simulink model "OFDM_Tx_HW"  (R2020a)
settings: Solver=FixedStepDiscrete  StartTime=0.0  StopTime=inf  RelTol=1e-3
PostLoadFcn:
  | run ./scripts/filter_setup;
InitFcn:
  | % Set parameters
  | fs = 1e6;
  | 
  | % Load all required variables
  | load('variables/read_addr_data');
  | load('variables/read_addr_cp');
  | load('variables/read_addr_pream');
  | load('variables/read_addr_rx');
  | load('variables/pilot');
  | load('variables/sc_index');
  | load('variables/LTSfreq');
  | load('variables/STSfreq');
  | load('variables/LTSread');
  | load('variables/STSread');
  | 
  | run ./scripts/rfgen;
undefined symbols (not defined in the file): CIC_fine_Rx
libraries: hdlsllib x13, dspsigops x5, dspmlti4 x3, xbsIndex_r4 x1, lib_ofdmrx x1, lib_ofdmtx x1, dspobslib x1, lib_interpolatetx x1
settings Model: SimulationMode=accelerator  Creator=njb13206  LastModifiedBy=LDM
settings OptimizationCC: BlockReduction=off  ConditionallyExecuteInputs=off  DefaultParameterBehavior=Inlined
settings DebuggingCC: AlgebraicLoopMsg=error  IntegerOverflowMsg=none  ParameterPrecisionLossMsg=none  IntegerSaturationMsg=none
settings HardwareCC: ProdBitPerPointer=32  ProdBitPerSizeT=32  ProdBitPerPtrDiffT=32  ProdLargestAtomicFloat=None  ProdIntDivRoundTo=Undefined  ProdEndianess=Unspecified  ProdWordSize=32  ProdHWDeviceType=ASIC/FPGA->ASIC/FPGA  TargetBitPerPointer=64  TargetBitPerSizeT=64  TargetBitPerPtrDiffT=64  TargetLongLongMode=on  TargetIntDivRoundTo=Zero  TargetEndianess=LittleEndian  TargetWordSize=64  TargetHWDeviceType=Custom Processor->MATLAB Host Computer  ProdEqTarget=off

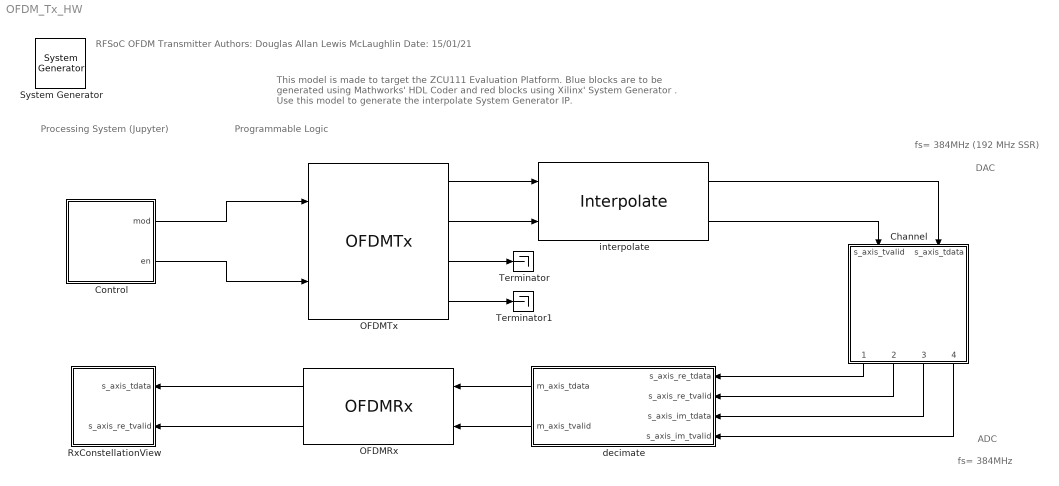
== system OFDM_Tx_HW ==
  note: This model is made to target the ZCU111 Evaluation Platform. Blue blocks are to be generated using Mathworks' HDL Coder and red blocks using Xilinx' System Generator .
      |
      | Use this model to generate the interpolate System Generator IP.
  note: Programmable Logic
  note: Processing System (Jupyter)
  note: DAC
  note: fs= 384MHz (192 MHz SSR)
  note: ADC
  note: fs= 384MHz
  note: RFSoC OFDM Transmitter
      | Authors: Douglas Allan
      | Lewis McLaughlin
      | Date: 15/01/21
  " System Generator" : xbsIndex_r4/ System Generator  Tag=genX  xilinxfamily=zynquplusRFSOC  part=xczu28dr  speed=-2-e  package=ffvg1517  synthesis_tool=Vivado  clock_wrapper=Clock Enables  directory=C:/Git/rfsoc_ofdm_workspace/models/sys_prj/tx  proj_type=Vivado  Synth_file=Vivado Synthesis Defaults  Impl_file=Vivado Implementation Defaults  testbench=off  simulink_period=1/192e6  sysclk_period=1000/192  dcm_input_clock_period=10  incr_netlist=off  trim_vbits=Everywhere in SubSystem  dbl_ovrd=According to Block Masks  core_generation=According to Block Masks  run_coregen=off  deprecated_control=off  eval_field=0  block_type=sysgen
  Channel : Subsystem
  Control : Subsystem  mask{mod_mask=512QAM, en=on}
      mask prompts: mod_mask "Modulation"; en "Enable"
      mask init:
      | % RF Signal Generator
      | if strcmpi(get_param(gcb, 'mod_mask'), 'BPSK')
      |     mod = 0;
      | elseif strcmpi(get_param(gcb, 'mod_mask'), 'QPSK')
      |     mod = 1;
      | elseif strcmpi(get_param(gcb, 'mod_mask'), '8PSK')
      |     mod = 2;
      | elseif strcmpi(get_param(gcb, 'mod_mask'), '16QAM')
      |     mod = 3;
      | elseif strcmpi(get_param(gcb, 'mod_mask'), '32QAM')
      |     mod = 4;
      | elseif strcmpi(get_param(gcb, 'mod_mask'), '64QAM')
      |     mod = 5;
      | elseif strcmpi(get_param(gcb, 'mod_mask'), '128QAM')
      |     mod = 6;
      | elseif strcmpi(get_param(gcb, 'mod_mask'), '256QAM')
      |     mod = 7;
      | elseif strcmpi(get_param(gcb, 'mod_mask'), '512QAM')
      |     mod = 8;
      | elseif strcmpi(get_param(gcb, 'mod_mask'), '1024QAM')
      |     mod = 9;
      | end
      mask TypeOptions mod_mask: BPSK | QPSK | 8PSK | 16QAM | 32QAM | 64QAM | 128QAM | 256QAM | 512QAM | 1024QAM
      mask DialogControl DescGroupVar Prompt: RF Signal Generator
      mask DialogControl DescTextVar Prompt: Exposes parameters the user can control from Jupyter when running on the target.
      mask DialogControl Container3 Prompt: Control
  OFDMRx : lib_ofdmrx/OFDMRx  SystemSampleTime=-1  Latency=0  AutoFrameSizeCalculation=off
  OFDMTx : lib_ofdmtx/OFDMTx  SystemSampleTime=-1  Latency=0  AutoFrameSizeCalculation=off
  RxConstellationView : Subsystem
  Terminator : Terminator
  Terminator1 : Terminator
  decimate : Subsystem
  interpolate : lib_interpolatetx/Interpolate  SystemSampleTime=-1  Latency=0  AutoFrameSizeCalculation=off
  wires:
  interpolate/1 -> Channel/2(s_axis_tdata)
  OFDMTx/1 -> interpolate/1
  OFDMTx/2 -> interpolate/2
  interpolate/2 -> Channel/1(s_axis_tvalid)
  Channel/4(m_axis_im_tvalid) -> decimate/4(s_axis_im_tvalid)
  OFDMRx/1 -> RxConstellationView/1(s_axis_tdata)
  OFDMRx/2 -> RxConstellationView/2(s_axis_re_tvalid)
  Channel/1(m00_axis_re_tdata) -> decimate/1(s_axis_re_tdata)
  Channel/2(m_axis_re_tvalid) -> decimate/2(s_axis_re_tvalid)
  Channel/3(m01_axis_im_tdata) -> decimate/3(s_axis_im_tdata)
  decimate/2(m_axis_tvalid) -> OFDMRx/2
  decimate/1(m_axis_tdata) -> OFDMRx/1
  Control/1(mod) -> OFDMTx/1
  Control/2(en) -> OFDMTx/2
  OFDMTx/3 -> Terminator/1
  OFDMTx/4 -> Terminator1/1

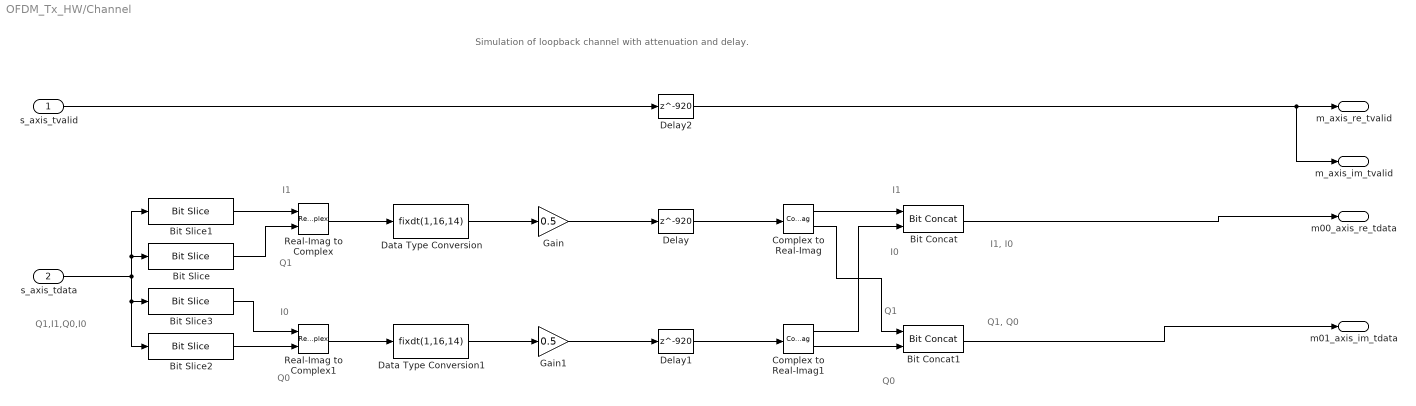
== system OFDM_Tx_HW/Channel ==
  note: Q1, Q0
  note: I1, I0
  note: Q0
  note: I0
  note: Q1
  note: I1
  note: Q1,I1,Q0,I0
  note: Simulation of loopback channel with attenuation and delay.
  note: I1
  note: I0
  note: Q1
  note: Q0
  s_axis_tvalid : Inport
  s_axis_tdata : Inport  Port=2
  Bit Concat : hdlsllib/Logic and Bit Operations/Bit Concat  numInputs=2
  Bit Concat1 : hdlsllib/Logic and Bit Operations/Bit Concat  numInputs=2
  Bit Slice : hdlsllib/Logic and Bit Operations/Bit Slice  lidx=63  ridx=48
      settings: SourceProductBaseCode=SL
  Bit Slice1 : hdlsllib/Logic and Bit Operations/Bit Slice  lidx=47  ridx=32
      settings: SourceProductBaseCode=SL
  Bit Slice2 : hdlsllib/Logic and Bit Operations/Bit Slice  lidx=31  ridx=16
      settings: SourceProductBaseCode=SL
  Bit Slice3 : hdlsllib/Logic and Bit Operations/Bit Slice  lidx=15  ridx=0
      settings: SourceProductBaseCode=SL
  Complex to Real-Imag : ComplexToRealImag
  Complex to Real-Imag1 : ComplexToRealImag
  Data Type Conversion : DataTypeConversion  OutDataTypeStr=fixdt(1,16,14)  ConvertRealWorld=Stored Integer (SI)
  Data Type Conversion1 : DataTypeConversion  OutDataTypeStr=fixdt(1,16,14)  ConvertRealWorld=Stored Integer (SI)
  Delay : Delay  DelayLength=920
  Delay1 : Delay  DelayLength=920
  Delay2 : Delay  DelayLength=920
  Gain : Gain  Gain=0.5  ParamDataTypeStr=double  OutDataTypeStr=fixdt(1,16,14)
  Gain1 : Gain  Gain=0.5  ParamDataTypeStr=double  OutDataTypeStr=fixdt(1,16,14)
  Real-Imag to Complex : RealImagToComplex
  Real-Imag to Complex1 : RealImagToComplex
  m00_axis_re_tdata : Outport  VectorParamsAs1DForOutWhenUnconnected=off
  m_axis_re_tvalid : Outport  Port=2  VectorParamsAs1DForOutWhenUnconnected=off
  m01_axis_im_tdata : Outport  Port=3  VectorParamsAs1DForOutWhenUnconnected=off
  m_axis_im_tvalid : Outport  Port=4  VectorParamsAs1DForOutWhenUnconnected=off
  wires:
  Gain/1 -> Delay/1
  s_axis_tvalid/1 -> Delay2/1
  Delay/1 -> Complex to Real-Imag/1
  s_axis_tdata/1 -> Bit Slice1/1, Bit Slice/1, Bit Slice2/1, Bit Slice3/1
  Delay1/1 -> Complex to Real-Imag1/1
  Gain1/1 -> Delay1/1
  Bit Concat/1 -> m00_axis_re_tdata/1
  Bit Concat1/1 -> m01_axis_im_tdata/1
  Bit Slice/1 -> Real-Imag to Complex/2
  Bit Slice1/1 -> Real-Imag to Complex/1
  Bit Slice2/1 -> Real-Imag to Complex1/2
  Bit Slice3/1 -> Real-Imag to Complex1/1
  Real-Imag to Complex/1 -> Data Type Conversion/1
  Real-Imag to Complex1/1 -> Data Type Conversion1/1
  Complex to Real-Imag1/1 -> Bit Concat/2
  Complex to Real-Imag/1 -> Bit Concat/1
  Complex to Real-Imag1/2 -> Bit Concat1/2
  Complex to Real-Imag/2 -> Bit Concat1/1
  Data Type Conversion/1 -> Gain/1
  Data Type Conversion1/1 -> Gain1/1
  Delay2/1 -> m_axis_im_tvalid/1, m_axis_re_tvalid/1

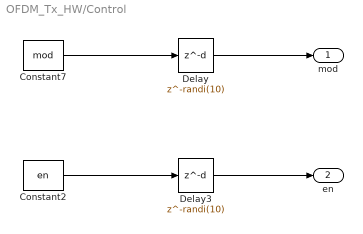
== system OFDM_Tx_HW/Control ==
  Constant2 : Constant  Value=en  OutDataTypeStr=boolean  SampleTime=1/(fs*12)
  Constant7 : Constant  Value=mod  VectorParams1D=off  OutDataTypeStr=uint32  SampleTime=1/(fs*12)
  Delay : Delay  DelayLength=randi(10)
  Delay3 : Delay  DelayLength=randi(10)
  mod : Outport  VectorParamsAs1DForOutWhenUnconnected=off
  en : Outport  Port=2  VectorParamsAs1DForOutWhenUnconnected=off
  wires:
  Constant2/1 -> Delay3/1
  Constant7/1 -> Delay/1
  Delay/1 -> mod/1
  Delay3/1 -> en/1

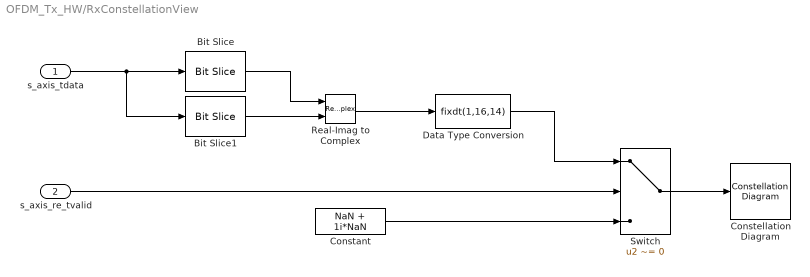
== system OFDM_Tx_HW/RxConstellationView ==
  s_axis_tdata : Inport
  s_axis_re_tvalid : Inport  Port=2
  Bit Slice : hdlsllib/Logic and Bit Operations/Bit Slice  lidx=15  ridx=0
      settings: SourceProductBaseCode=SL
  Bit Slice1 : hdlsllib/Logic and Bit Operations/Bit Slice  lidx=31  ridx=16
      settings: SourceProductBaseCode=SL
  Constant : Constant  Value=NaN + 1i*NaN  OutDataTypeStr=double  SampleTime=-1
  Constellation Diagram : ConstellationDiagram
  Data Type Conversion : DataTypeConversion  OutDataTypeStr=fixdt(1,16,14)  ConvertRealWorld=Stored Integer (SI)
  Real-Imag to Complex : RealImagToComplex
  Switch : Switch  Criteria=u2 ~= 0
  wires:
  Switch/1 -> Constellation Diagram/1
  Constant/1 -> Switch/3
  s_axis_re_tvalid/1 -> Switch/2
  Real-Imag to Complex/1 -> Data Type Conversion/1
  Bit Slice/1 -> Real-Imag to Complex/1
  s_axis_tdata/1 -> Bit Slice1/1, Bit Slice/1
  Bit Slice1/1 -> Real-Imag to Complex/2
  Data Type Conversion/1 -> Switch/1

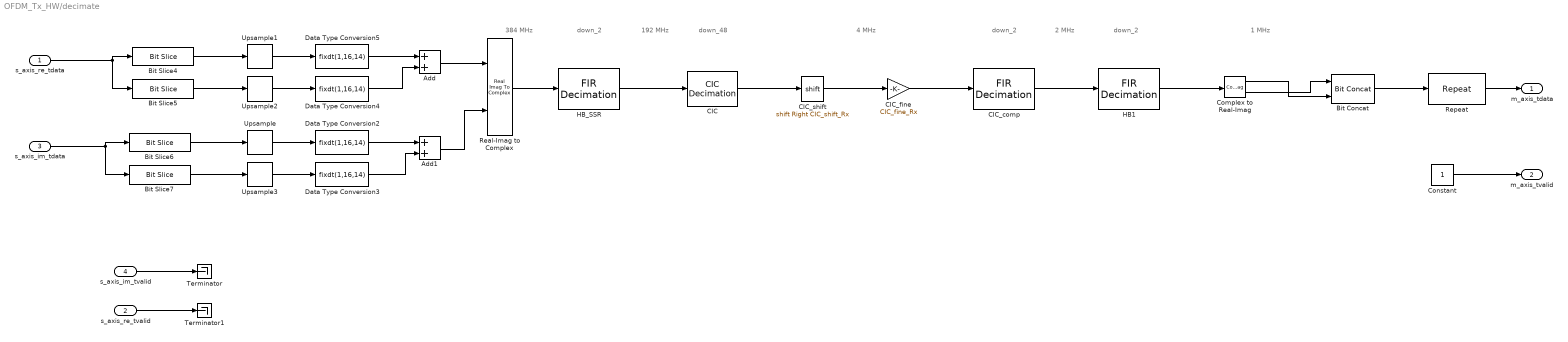
== system OFDM_Tx_HW/decimate ==
  note: down_2
  note: 2 MHz
  note: 4 MHz
  note: 192 MHz
  note: 384 MHz
  note: 1 MHz
  note: down_48
  note: down_2
  note: down_2
  s_axis_re_tdata : Inport
  s_axis_re_tvalid : Inport  Port=2
  s_axis_im_tdata : Inport  Port=3
  s_axis_im_tvalid : Inport  Port=4
  Add : Sum  OutDataTypeStr=fixdt(1,16,14)
  Add1 : Sum  OutDataTypeStr=fixdt(1,16,14)
  Bit Concat : hdlsllib/Logic and Bit Operations/Bit Concat  numInputs=2
  Bit Slice4 : hdlsllib/Logic and Bit Operations/Bit Slice  lidx=15  ridx=0
      settings: SourceProductBaseCode=SL
  Bit Slice5 : hdlsllib/Logic and Bit Operations/Bit Slice  lidx=31  ridx=16
      settings: SourceProductBaseCode=SL
  Bit Slice6 : hdlsllib/Logic and Bit Operations/Bit Slice  lidx=15  ridx=0
      settings: SourceProductBaseCode=SL
  Bit Slice7 : hdlsllib/Logic and Bit Operations/Bit Slice  lidx=31  ridx=16
      settings: SourceProductBaseCode=SL
  CIC : dspobslib/CIC Decimation  filtFrom=Multirate object in workspace  filtobj=CIC_Rx  ftype=Decimator  R=2  M=1  N=2  filterInternals=Full precision  BPS=[16 16 16 16]  FLPS=0  outputWordLength=32  outputFracLength=0  launchFVT=off  framing=Maintain input frame rate  RateOptions=Allow multirate processing
      settings: SourceProductBaseCode=DS
  CIC_comp : dspmlti4/FIR Decimation  FilterSource=Dialog parameters  h=WComp_Rx.Numerator  D=2  filtStruct=Direct form  FilterObject=FDECIM  framing=Allow multirate processing  inputOffset=0  outputBufInitCond=0  roundingMode=Floor  overflowMode=off  firstCoeffMode=Binary point scaling  firstCoeffWordLength=16  firstCoeffFracLength=15  firstCoeffDataTypeStr=fixdt(1,16,15)  firstCoeffMin=[]  firstCoeffMax=[]  firstCoeffLastDataTypeStr=fixdt(1,16,15)  outputMode=Binary point scaling  outputWordLength=16  outputFracLength=14  outputDataTypeStr=fixdt(1,16,14)  outputMin=[]  outputMax=[]  outputLastDataTypeStr=fixdt(1,16,14)
  CIC_fine : Gain  Gain=CIC_fine_Rx  OutDataTypeStr=fixdt(1,16,14)
  CIC_shift : ArithShift  BitShiftNumber=CIC_shift_Rx  BitShiftDirection=Right
  Complex to Real-Imag : ComplexToRealImag
  Constant : Constant  OutDataTypeStr=boolean  SampleTime=1/(fs*12)
  Data Type Conversion{2..5} (4 alike) : DataTypeConversion  OutDataTypeStr=fixdt(1,16,14)  ConvertRealWorld=Stored Integer (SI)
  HB1 : dspmlti4/FIR Decimation  FilterSource=Dialog parameters  h=W_HB.Numerator  D=2  filtStruct=Direct form  FilterObject=FDECIM  framing=Allow multirate processing  inputOffset=0  outputBufInitCond=0  roundingMode=Floor  overflowMode=off  firstCoeffMode=Binary point scaling  firstCoeffWordLength=16  firstCoeffFracLength=15  firstCoeffDataTypeStr=fixdt(1,16,15)  firstCoeffMin=[]  firstCoeffMax=[]  firstCoeffLastDataTypeStr=fixdt(1,16,15)  outputMode=Binary point scaling  outputWordLength=16  outputFracLength=14  outputDataTypeStr=fixdt(1,16,14)  outputMin=[]  outputMax=[]  outputLastDataTypeStr=fixdt(1,16,14)
  HB_SSR : dspmlti4/FIR Decimation  FilterSource=Dialog parameters  h=W_HB.Numerator  D=2  filtStruct=Direct form  FilterObject=FDECIM  framing=Allow multirate processing  inputOffset=0  outputBufInitCond=0  roundingMode=Floor  overflowMode=off  firstCoeffMode=Binary point scaling  firstCoeffWordLength=16  firstCoeffFracLength=15  firstCoeffDataTypeStr=fixdt(1,16,15)  firstCoeffMin=[]  firstCoeffMax=[]  firstCoeffLastDataTypeStr=fixdt(1,16,15)  outputMode=Binary point scaling  outputWordLength=16  outputFracLength=14  outputDataTypeStr=fixdt(1,16,14)  outputMin=[]  outputMax=[]  outputLastDataTypeStr=fixdt(1,16,14)
  Real-Imag to Complex : RealImagToComplex
  Repeat : dspsigops/Repeat  N=12  InputProcessing=Columns as channels (frame based)  RateOptions=Allow multirate processing  ic=0  mode=Unused parameter value
  Terminator : Terminator
  Terminator1 : Terminator
  Upsample : dspsigops/Upsample  N=2  phase=0  RateOptions=Allow multirate processing  ic=0  mode=Unused parameter value
  Upsample1 : dspsigops/Upsample  N=2  phase=0  RateOptions=Allow multirate processing  ic=0  mode=Unused parameter value
  Upsample2 : dspsigops/Upsample  N=2  phase=1  RateOptions=Allow multirate processing  ic=0  mode=Unused parameter value
  Upsample3 : dspsigops/Upsample  N=2  phase=1  RateOptions=Allow multirate processing  ic=0  mode=Unused parameter value
  m_axis_tdata : Outport
  m_axis_tvalid : Outport  Port=2
  wires:
  CIC_comp/1 -> HB1/1
  CIC_shift/1 -> CIC_fine/1
  HB_SSR/1 -> CIC/1
  CIC/1 -> CIC_shift/1
  CIC_fine/1 -> CIC_comp/1
  HB1/1 -> Complex to Real-Imag/1
  Real-Imag to Complex/1 -> HB_SSR/1
  s_axis_im_tvalid/1 -> Terminator/1
  s_axis_re_tvalid/1 -> Terminator1/1
  Repeat/1 -> m_axis_tdata/1
  Data Type Conversion3/1 -> Add1/2
  Data Type Conversion5/1 -> Add/1
  Upsample2/1 -> Data Type Conversion4/1
  Upsample3/1 -> Data Type Conversion3/1
  Data Type Conversion4/1 -> Add/2
  Bit Slice7/1 -> Upsample3/1
  Bit Slice6/1 -> Upsample/1
  Upsample/1 -> Data Type Conversion2/1
  Add/1 -> Real-Imag to Complex/1
  Bit Slice5/1 -> Upsample2/1
  Data Type Conversion2/1 -> Add1/1
  s_axis_re_tdata/1 -> Bit Slice4/1, Bit Slice5/1
  Add1/1 -> Real-Imag to Complex/2
  s_axis_im_tdata/1 -> Bit Slice6/1, Bit Slice7/1
  Upsample1/1 -> Data Type Conversion5/1
  Bit Slice4/1 -> Upsample1/1
  Complex to Real-Imag/1 -> Bit Concat/2
  Complex to Real-Imag/2 -> Bit Concat/1
  Bit Concat/1 -> Repeat/1
  Constant/1 -> m_axis_tvalid/1
